simulink model "FeedbackLinearizationController"  (R2019b)
settings: Solver=VariableStepAuto  StartTime=0.0  StopTime=50  RelTol=1e-3
undefined symbols (not defined in the file): B, b1, b2, C, D, gravity, l, q0
settings Model: Creator=ariannagasparri  LastModifiedBy=ariannagasparri

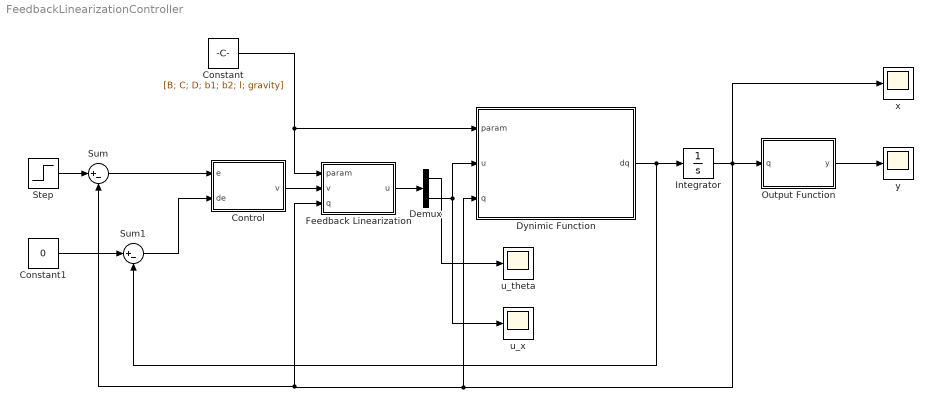
== system FeedbackLinearizationController ==
  Constant : Constant  Value=[B; C; D; b1; b2; l; gravity]
  Constant1 : Constant  Value=0
  Control : MATLAB Function  TreatAsAtomicUnit=on
  Demux : Demux  Outputs=2
  Dynimic Function : MATLAB Function  TreatAsAtomicUnit=on
  Feedback Linearization : MATLAB Function  TreatAsAtomicUnit=on
  Integrator : Integrator  InitialCondition=q0
  Output Function : MATLAB Function  TreatAsAtomicUnit=on
  Step : Step  SampleTime=0
  Sum : Sum  Inputs=|+-
  Sum1 : Sum  Inputs=|+-
  u_theta : Scope
  u_x : Scope
  x : Scope
  y : Scope
  wires:
  Dynimic Function/1(dq) -> Sum1/2, Integrator/1
  Integrator/1 -> Dynimic Function/3(q), Sum/2, Feedback Linearization/3(q), x/1, Output Function/1(q)
  Constant/1 -> Feedback Linearization/1(param), Dynimic Function/1(param)
  Demux/1 -> u_theta/1
  Demux/2 -> Dynimic Function/2(u), u_x/1
  Feedback Linearization/1(u) -> Demux/1
  Sum/1 -> Control/1(e)
  Step/1 -> Sum/1
  Output Function/1(y) -> y/1
  Control/1(v) -> Feedback Linearization/2(v)
  Constant1/1 -> Sum1/1
  Sum1/1 -> Control/2(de)

== matlab function FeedbackLinearizationController/Feedback Linearization ==
  data: param input; v input; u output; q input
function u = fcn(param, v, q)

u = zeros(2,1);

B = param(1);
C = param(2);
D = param(3);
b1 = param(4);
b2 = param(5);
l = param(6);
gravity = param(7);

u(1) = (v(1) - Lf2h1_fun(B,C,D,b1,b2,gravity,l,q)) / LgLfh1_fun(B,C,D,l,q);
u(2) = (v(2) - Lf2h2_fun(B,C,b2,gravity,l,q)) / LgLfh2_fun(B,C,D,l,q);

end

== matlab function FeedbackLinearizationController/Dynimic Function ==
  data: param input; u input; dq output; q input
function dq = fcn(param, u, q)

B = param(1);
C = param(2);
D = param(3);
b1 = param(4);
b2 = param(5);
l = param(6);
gravity = param(7);

dq = f_fun(B,C,D,b1,b2,gravity,l,q) + g_fun(B,C,D,l,q)*u;

end

== matlab function FeedbackLinearizationController/Output Function ==
  data: q input; y output
function y = fcn(q)

y = h_fun(q);

end

== matlab function FeedbackLinearizationController/Control ==
  data: e input; v output; de input
function v = fcn(e, de)

kp = 100;
kd = 10;

v = kp * e + kd * de;

end
